simulink model "Simulink_Model"  (R2021a)
settings: Solver=VariableStepAuto  StartTime=0.0  StopTime=inf  FixedStep=1  RelTol=1e-3
model workspace (MAT data in the model file):
  M = 1200
  R = 1
libraries: pid_lib x1
settings Model: EnablePacing=on  Creator=matteopenlington  LastModifiedBy=matteopenlington
settings DebuggingCC: UnderSpecifiedDimensionMsg=warning

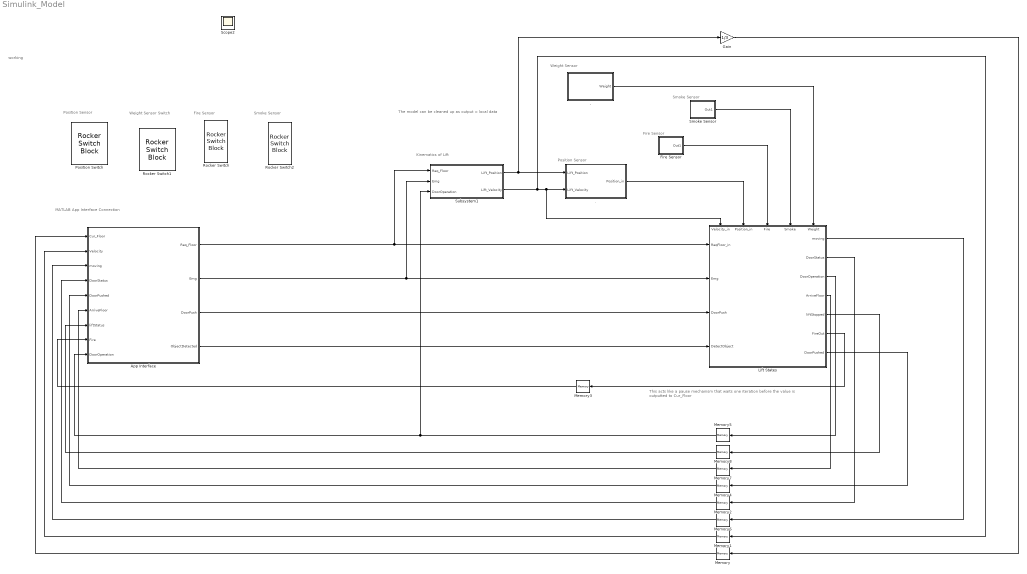
== system Simulink_Model ==
  note: working
  note: MATLAB App Interface Connection
  note: Fire Sensor
  note: Smoke Sensor
  note: Kinematics of Lift
  note: The model can be cleaned up as output = local data
  note: This acts like a pause mechanism that
      | waits one iteration before the value is
      | outputted to Cur_Floor
  note: Weight Sensor Switch
  note: Weight Sensor
  note: Position Sensor
  note: Position Sensor
  note: Fire Sensor
  note: Smoke Sensor
  , : Subsystem
  . : Subsystem
  App Interface : Stateflow chart  TreatAsAtomicUnit=on
      settings: PortSchema="{\"entries\":[{\"content\":{\"sides\":[{\"content\":{\"connectorIds\":[\"In1\",\"In2\",\"In6\",\"In3\",\"In4\",\"In7\",\"In9\",\"In8\",\"In5\"]},\"type\":\"ConnectorPlacement.EquallySpacedRectSide\",\"uuid\":\"ef86dee1-50cd-47ea-bc75-e3c16101b464\"},{\"content\":{\"connectorIds\":[\"Out1\",\"Out2\",\"Out3\",\"Out4\"],\"side\":\"RIGHT\"},\"type\":\"ConnectorPlacement.EquallySpacedRectSide\",\"uuid\":\"2ba459ed-9838-4da4-8149-392158b3da7c\"},{\"content\":{\"connectorIds\":[],\"side\":\"TOP\"},\"type\":\"ConnectorPlacement.EquallySpacedRectSide\",\"uuid\":\"d04a1450-e40a-42c5-8ca5-ab8bc8570c42\"}]},\"type\":\"ConnectorPlacement.EquallySpacedConnector\",\"uuid\":\"548c1efd-1acc-447b-a5db-88314a01fdab\"}],\"packageUris\":[\"http://schema.mathworks.com/mf0/Connector/R2020b\"],\"version\":\"1.0\"}"
  Fire Sensor : Subsystem
  Gain : Gain  Gain=1/3
  Lift States : Stateflow chart  TreatAsAtomicUnit=on
      settings: PortSchema="{\"entries\":[{\"content\":{\"sides\":[{\"content\":{\"connectorIds\":[\"In1\",\"In5\",\"In6\",\"In7\"]},\"type\":\"ConnectorPlacement.EquallySpacedRectSide\",\"uuid\":\"bd67e075-ced7-4894-beb9-3d24b34d513a\"},{\"content\":{\"connectorIds\":[\"Out1\",\"Out2\",\"Out4\",\"Out5\",\"Out6\",\"Out7\",\"Out3\"],\"side\":\"RIGHT\"},\"type\":\"ConnectorPlacement.EquallySpacedRectSide\",\"uuid\":\"62974800-2f1d-440c-84a5-b13d0b321f49\"},{\"content\":{\"connectorIds\":[\"In9\",\"In8\",\"In3\",\"In4\",\"In2\"],\"side\":\"TOP\"},\"type\":\"ConnectorPlacement.EquallySpacedRectSide\",\"uuid\":\"b0ebe389-7aaa-432d-aca6-247e3589a149\"}]},\"type\":\"ConnectorPlacement.EquallySpacedConnector\",\"uuid\":\"bed4184c-0ba6-4939-b370-ce80092994a7\"}],\"packageUris\":[\"http://schema.mathworks.com/mf0/Connector/R2020b\"],\"version\":\"1.0\"}"
  Memory{,1..8} (9 alike) : Memory
  Position Switch : RockerSwitchBlock
      settings: Values={{'Off', 'On'}, [0 1]}
  Rocker Switch : RockerSwitchBlock
      settings: Values={{'Off', 'On'}, [0 1]}
  Rocker Switch1 : RockerSwitchBlock
      settings: Values={{'Off', 'On'}, [0 1]}
  Rocker Switch2 : RockerSwitchBlock
      settings: Values={{'Off', 'On'}, [0 1]}
  Smoke Sensor : Subsystem
  Subsystem1 : Subsystem
  Scope2 : Scope
  wires:
  ./1(Position_in) -> Lift States/8(Position_in)
  Memory2/1 -> App Interface/3(DoorStatus)
  App Interface/4(ObjectDetected) -> Lift States/7(DetectObject)
  Memory4/1 -> App Interface/4(DoorPushed)
  Lift States/4(DoorOperation) -> Memory5/1
  Lift States/3(DoorPushed) -> Memory4/1
  Memory/1 -> App Interface/1(Cur_Floor)
  Memory6/1 -> App Interface/6(moving)
  Lift States/5(ArriveFloor) -> Memory7/1
  Subsystem1/1(Lift_Position) -> ./1(Lift_Position), Gain/1
  Subsystem1/2(Lift_Velocity) -> ./2(Lift_Velocity), Lift States/9(Velocity_in), Memory1/1
  Lift States/2(DoorStatus) -> Memory2/1
  Memory5/1 -> Subsystem1/3(DoorOperation), App Interface/5(DoorOperation)
  Lift States/1(moving) -> Memory6/1
  App Interface/3(DoorPush) -> Lift States/6(DoorPush)
  ,/1(Weight) -> Lift States/2(Weight)
  Memory1/1 -> App Interface/2(Velocity)
  Gain/1 -> Memory/1
  App Interface/2(Emg) -> Subsystem1/2(Emg), Lift States/5(Emg)
  App Interface/1(Req_Floor) -> Subsystem1/1(Req_Floor), Lift States/1(ReqFloor_in)
  Memory7/1 -> App Interface/7(ArriveFloor)
  Fire Sensor/1(Out1) -> Lift States/3(Fire)
  Smoke Sensor/1(Out1) -> Lift States/4(Smoke)
  Lift States/6(liftStopped) -> Memory8/1
  Memory8/1 -> App Interface/9(liftStatus)
  Lift States/7(FireOut) -> Memory3/1
  Memory3/1 -> App Interface/8(Fire)

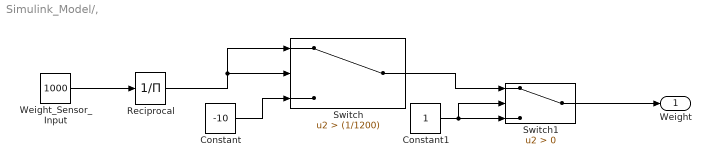
== system Simulink_Model/, ==
  Constant : Constant  Value=-10
  Constant1 : Constant
  Reciprocal : Product  Inputs=/
  Switch : Switch  Criteria=u2 > Threshold  Threshold=(1/1200)
  Switch1 : Switch  Criteria=u2 > Threshold
  Weight_Sensor_Input : Constant  Value=1000
  Weight : Outport
  wires:
  Weight_Sensor_Input/1 -> Reciprocal/1
  Switch/1 -> Switch1/1
  Constant/1 -> Switch/3
  Constant1/1 -> Switch1/3, Switch1/2
  Switch1/1 -> Weight/1
  Reciprocal/1 -> Switch/1, Switch/2

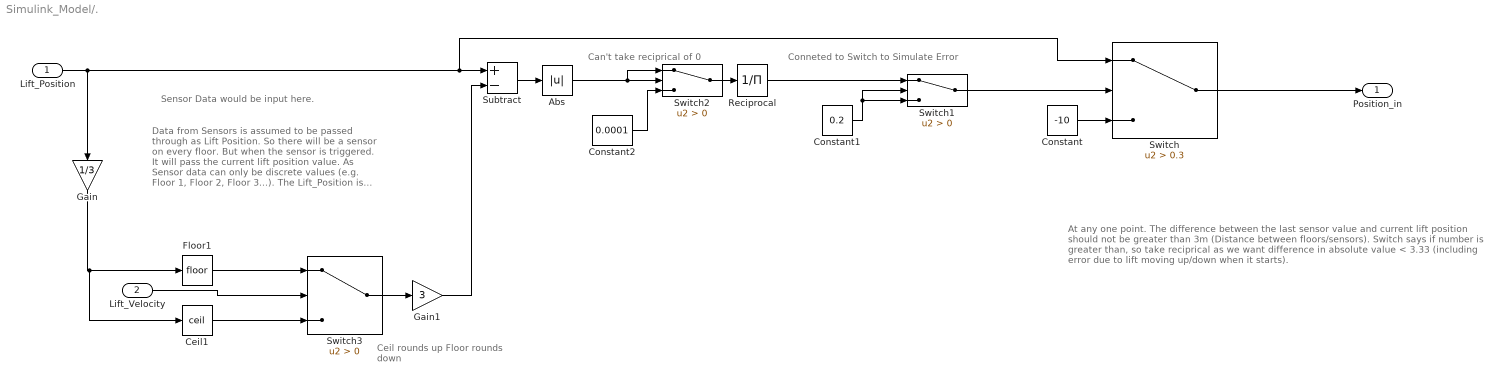
== system Simulink_Model/. ==
  note: Can't take reciprical of 0
  note: At any one point. The difference between the last sensor value and current lift position should not be greater than 3m (Distance between floors/sensors).
      |
      | Switch says if number is greater than, so take reciprical as we want difference in absolute value < 3.33 (including error due to lift moving up/down when it starts).
  note: Ceil rounds up
      | Floor rounds down
  note: Data from Sensors is assumed to be passed through as Lift Position. So there will be a sensor on every floor. But when the sensor is triggered. It will pass the current lift position value.
      |
      | As Sensor data can only be discrete values (e.g. Floor 1, Floor 2, Floor 3...). The Lift_Position is rounded to the integer according to whether velocity is up or down, as the opposite will be where the last stop was.
  note: Sensor Data would be input here.
  note: Conneted to Switch to Simulate Error
  Lift_Position : Inport
  Lift_Velocity : Inport  Port=2
  Abs : Abs
  Ceil1 : Rounding  Operator=ceil
  Constant : Constant  Value=-10
  Constant1 : Constant  Value=0.2
  Constant2 : Constant  Value=0.0001
  Floor1 : Rounding
  Gain : Gain  Gain=1/3
  Gain1 : Gain  Gain=3
  Reciprocal : Product  Inputs=/
  Subtract : Sum  Inputs=+-
  Switch : Switch  Criteria=u2 > Threshold  Threshold=0.3
  Switch1 : Switch  Criteria=u2 > Threshold
  Switch2 : Switch  Criteria=u2 > Threshold
  Switch3 : Switch  Criteria=u2 > Threshold
  Position_in : Outport
  wires:
  Lift_Position/1 -> Subtract/1, Switch/1, Gain/1
  Subtract/1 -> Abs/1
  Constant/1 -> Switch/3
  Switch/1 -> Position_in/1
  Switch1/1 -> Switch/2
  Abs/1 -> Switch2/1, Switch2/2
  Constant1/1 -> Switch1/3, Switch1/2
  Lift_Velocity/1 -> Switch3/2
  Switch3/1 -> Gain1/1
  Floor1/1 -> Switch3/1
  Ceil1/1 -> Switch3/3
  Gain/1 -> Floor1/1, Ceil1/1
  Gain1/1 -> Subtract/2
  Constant2/1 -> Switch2/3
  Switch2/1 -> Reciprocal/1
  Reciprocal/1 -> Switch1/1

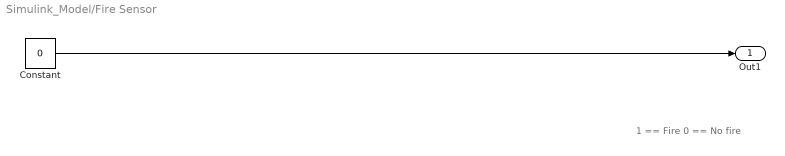
== system Simulink_Model/Fire Sensor ==
  note: 1 == Fire
      | 0 == No fire
  Constant : Constant  Value=0
  Out1 : Outport
  wires:
  Constant/1 -> Out1/1

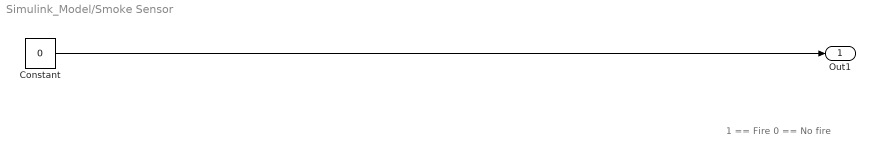
== system Simulink_Model/Smoke Sensor ==
  note: 1 == Fire
      | 0 == No fire
  Constant : Constant  Value=0
  Out1 : Outport
  wires:
  Constant/1 -> Out1/1

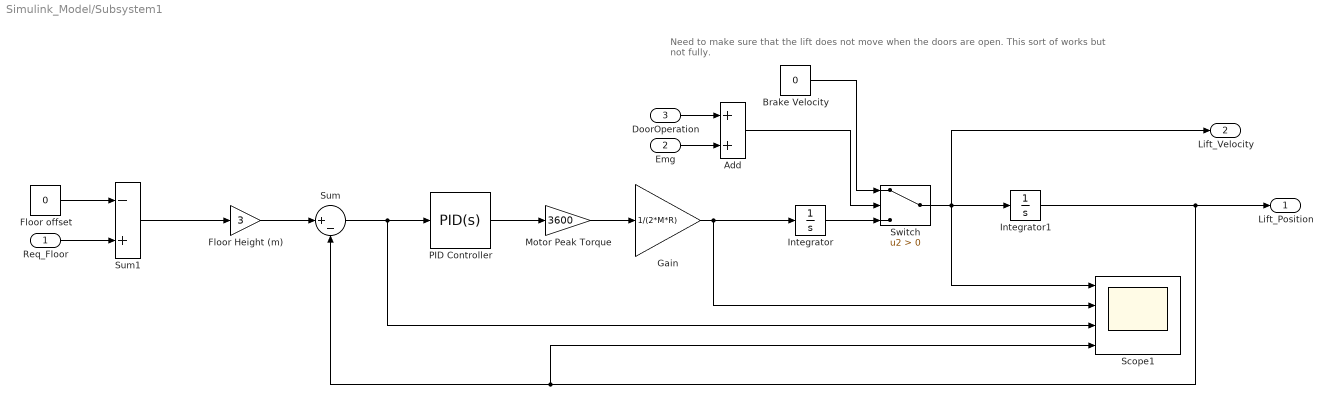
== system Simulink_Model/Subsystem1 ==
  note: Need to make sure that the lift does not move when the doors are open. This sort of works but not fully.
  Req_Floor : Inport
  Emg : Inport  Port=2
  DoorOperation : Inport  Port=3
  Add : Sum
  Brake Velocity : Constant  Value=0
  Floor Height (m) : Gain  Gain=3
  Floor offset : Constant  Value=0
  Gain : Gain  Gain=1/(2*M*R)
  Integrator : Integrator
  Integrator1 : Integrator
  Motor Peak Torque : Gain  Gain=3600
  PID Controller : pid_lib/PID Controller  Controller=PID  Form=Parallel  TimeDomain=Continuous-time  UseExternalTs=off  SampleTime=-1  IntegratorMethod=Forward Euler  FilterMethod=Forward Euler  ControllerParametersSource=internal  P=1  I=0  D=2  UseFilter=on  N=5.45  TunerSelectOption=Transfer Function Based (PID Tuner App)  InitialConditionSource=internal  InitialConditionForIntegrator=0  InitialConditionForFilter=0  DifferentiatorICPrevScaledInput=0  ExternalReset=none  TrackingMode=off  Kt=1  LimitOutput=on  SatLimitsSource=internal  UpperSaturationLimit=1  LowerSaturationLimit=-1  LinearizeAsGain=on  AntiWindupMode=none  Kb=1  POutMin=[]  POutMax=[]  IOutMin=[]  IOutMax=[]  DOutMin=[]  DOutMax=[]  NOutMin=[]  NOutMax=[]  SumOutMin=[]  SumOutMax=[]  SaturationOutMin=[]  SaturationOutMax=[]  PParamMin=[]  PParamMax=[]  IParamMin=[]  IParamMax=[]  DParamMin=[]  DParamMax=[]  NParamMin=[]  NParamMax=[]  KbParamMin=[]  KbParamMax=[]  KtParamMin=[]  KtParamMax=[]  KbOutMin=[]  KbOutMax=[]  KtOutMin=[]  KtOutMax=[]  IntegratorOutMin=[]  IntegratorOutMax=[]  FilterOutMin=[]  FilterOutMax=[]  SumI1OutMin=[]  SumI1OutMax=[]  SumI2OutMin=[]  SumI2OutMax=[]  SumI3OutMin=[]  SumI3OutMax=[]  SumI4OutMin=[]  SumI4OutMax=[]  SumDOutMin=[]  SumDOutMax=[]  DifferentiatorOutMin=[]  DifferentiatorOutMax=[]  FilterDiffOutCoefMin=[]  FilterDiffOutCoefMax=[]  ReciprocalOutMin=[]  ReciprocalOutMax=[]  SumDenOutMin=[]  SumDenOutMax=[]  SumNumOutMin=[]  SumNumOutMax=[]  DivideOutMin=[]  DivideOutMax=[]  UdiffTsProdOutMin=[]  UdiffTsProdOutMax=[]  NTsProdOutMin=[]  NTsProdOutMax=[]  UintegralTsProdOutMin=[]  UintegralTsProdOutMax=[]  UngainTsProdOutMin=[]  UngainTsProdOutMax=[]  IntegratorContinuousStateAttributes=''  IntegratorStateMustResolveToSignalObject=off  IntegratorRTWStateStorageClass=Auto  FilterContinuousStateAttributes=''  FilterStateMustResolveToSignalObject=off  FilterRTWStateStorageClass=Auto  ParallelPVariant=InternalParameters  IdealPVariant=Disabled  IVariant=InternalParameters  DVariant=InternalParameters  IntegratorVariant=Continuous  SatVariant=Enabled  AWVariant=Passthrough  PCopyVariant=Disabled  TRVariant=Disabled  FdbkBlocksVariant=Forward  IdealPFdbkVariant=Disabled  SatFdbkVariant=Disabled  DerivativeFilterVariant=ContFilter  NVariant=InternalParameters  NCopyVariant=Disabled  FilterICVariant=InternalICsFilter  IntegratorICVariant=InternalICs  ExternalResetVariant=Disabled  TRSumVariant=Passthrough  SumFdbkVariant=Disabled  SumVariant=Sum_PID  TsampFilterVariant=InternalTs  TsampNgainVariant=Passthrough  TsampIntegralVariant=Passthrough  ExternalSaturationOutDataTypeStr=Inherit: Same as second input
  Scope1 : Scope  NumInputPorts=4
  Sum : Sum  Inputs=|+-
  Sum1 : Sum  Inputs=-+
  Switch : Switch  Criteria=u2 > Threshold
  Lift_Position : Outport
  Lift_Velocity : Outport  Port=2
  wires:
  Req_Floor/1 -> Sum1/2
  Gain/1 -> Scope1/2, Integrator/1
  Sum/1 -> Scope1/3, PID Controller/1
  PID Controller/1 -> Motor Peak Torque/1
  Floor Height (m)/1 -> Sum/1
  Sum1/1 -> Floor Height (m)/1
  Integrator/1 -> Switch/3
  Integrator1/1 -> Lift_Position/1, Scope1/4, Sum/2
  Motor Peak Torque/1 -> Gain/1
  Floor offset/1 -> Sum1/1
  Switch/1 -> Scope1/1, Lift_Velocity/1, Integrator1/1
  Brake Velocity/1 -> Switch/1
  Emg/1 -> Add/2
  DoorOperation/1 -> Add/1
  Add/1 -> Switch/2

== stateflow chart Simulink_Model/App Interface ==
  state InterfaceFromApp
    en:
    coder.extrinsic('AppWSimulink', 'updateCounter', 'Emergency', 'DoorOperationReq', 'updateDoorStatus', 'CallDirection', 'liftCall', 'DetectObject', 'liftStopped', 'FireFnc', 'checkPassengerMatrix');
    app = AppWSimulink(this);
    initialiseData();
    Emergency(app,Emg);
    DoorOperationReq(app, DoorPush);
    %liftCall(app, Velocity, Cur_Floor);
    du:
    if hasChanged(Cur_Floor)
    updateCounter(app, Cur_Floor, moving, DoorOperation);
    end
    if abs(Req_Floor - Cur_Floor) < 0.1
    updateDoorStatus(app,DoorStatus, Cur_Floor, ArriveFloor);
    end
    if (Emg == 1)
    Reset;
    end
    if DoorPushed == 1
    DoorPush = -2;
    end
    if DoorOperation == 0
    end
    DetectObject(app);
    if DoorOperation == 1
    Req_Floor = Cur_Floor;
    end
    if liftStatus == 1 && ifRequested == 1
    liftStopped(app);
    end
    if Fire == 1
    %FireFnc(app)
    end
    if moving == 1
    ifRequested = 0;
    end
    % checkPassengerMatrix(app)
    liftDesination = Req_Floor;
    state initialiseData [function]
      (default) -> (junction 12) : {
          | %CurFloor = 0;
          | Req_Floor = 1;
          | Emg = 0;
          | DoorPush =-2;
          | ObjectDetected =0;
          | ifRequested = 0;
          | }
    state Reset [function]
      (default) -> (junction 119) : {
          | Req_Floor = Cur_Floor;
          | DoorPush =3;
          | }
  (default) -> InterfaceFromApp
  data: app local; Cur_Floor input; Req_Floor output; Emg output; Velocity input; DoorPush output; DoorStatus input; ObjectDetected output; DoorPushed input; DoorOperation input; moving input; ArriveFloor input; Fire input; liftStatus input; liftDesination local; ifRequested local

== stateflow chart Simulink_Model/Lift States ==
  state No_Error2
    en:
    initialiseData;
    state initialiseData [function]
      (default) -> (junction 330) : {door = 0;
          | doorClose = 0;
          | hasOpened = 1;
          | ArriveFloor = 0;
          | DoorStatus = 3;
          | DoorOperation = 0;
          | DoorPushed = 0;
          | }
    state Motion [group]
      state MovingUp
        entry:
        moving = 1;
        liftStopped = 0;
        hasOpened =0;
        exit:
        moving = 0;
      state MovingDown
        entry:
        moving = 2;
        liftStopped = 0;
        hasOpened = 0;
        exit:
        moving =0;
    state Not_Moving
      entry:
      Cur_Floor;
      NxtFloor;
      liftStopped = 1;
      state NxtFloor [function]
        (default) -> (junction 212)
        (junction 212) -> (junction 213) [order 1] : [isempty(ReqFloor_in)]{ReqFloor = -10}
        (junction 212) -> (junction 214) [order 2] : {ReqFloor = ReqFloor_in;}
        (junction 213) -> (junction 215)
        (junction 214) -> (junction 215)
      state Idle
        en:
      state Doors
        note: Value of door isn't always 0 or 1
            |
            | Object Detection is always running whilst open. Value is simulated through app interface button.
        state OpOpening [function]
          note: If the door movement was simulated that value would end up being exactly 0 or 1. Because of step iterations you end up with 1.1 and -0.1. But the transitions account for this.
          (default) -> (junction 231) : [door <= 1]{door = door + 0.1;}
        state DoorOpening
          en:
          door = 0;
          doorClose = 0;
          DoorStatus = 0;
          du:
          OpOpening;
        state OpClosing [function]
          (default) -> (junction 244) : {door = door - 0.1;}
        state DoorClosing
          en:
          DoorStatus = 2;
          DoorPushed = 0;
          du:
          OpClosing;
        state DoorOpen
          entry:
          DoorStatus = 1;
          hasOpened = 1;
        state DoorClosed
          entry:
          DoorStatus =3;
          pause(2);
          doorClose = 1;
        (junction 318) -> DoorOpening
        DoorClosing -> (junction 318) [order 1] : [DetectObject == 1]
        (junction 321) -> DoorOpening
        DoorClosing -> (junction 321) [order 2] : [DoorPush == 0]{DoorPushed = 1;}
        DoorOpening -> DoorOpen : [door >= 1]{DoorPushed = 0;}
        DoorOpen -> DoorClosing [order 2] : [DoorPush == 1 && DetectObject == 0]{DoorPushed = 1;}
        DoorClosing -> DoorClosed [order 3] : [door <= 0]
        DoorOpen -> DoorClosing [order 1] : after(2,sec)[DetectObject == 0]
      (default) -> Idle
      Idle -> DoorOpening [order 1] : [ (ReqFloor - CurFloor)<0.01 && hasOpened == 0]{DoorOperation =1;, ArriveFloor=1;}
    state Cur_Floor [function]
      (default) -> (junction 279) : {CurFloor = (Position_in/3);}
    note: Set DoorPush == -2 because it has been completed. But don't want to set ObjectDetected == 0 because we need to run again and make sure there are no objects in the way.
    (default) -> Not_Moving
    Not_Moving -> MovingUp [order 1] : [Velocity_in > 0.2 && DoorOperation == 0]
    MovingUp -> Not_Moving : [abs(Velocity_in) < 0.01]
    Idle -> (junction 192) [order 2]
    (junction 192) -> (junction 193)
    Not_Moving -> MovingDown [order 2] : [Velocity_in < -0.2 && DoorOperation == 0]
    (junction 193) -> Not_Moving : after(1,sec)
    (junction 194) -> (junction 193)
    MovingDown -> Not_Moving : [abs(Velocity_in) < 0.01]
    Doors -> (junction 194) : [doorClose == 1]{DoorOperation = 0;, ArriveFloor = 0;}
  state Error_States
    en:
    state Emergency
      en:
      DoorStatus = 3;
      hasOpened = 0;
      moving = 0;
    state Position_Sensor
      en:
      DoorStatus = 0;
      hasOpened = 0;
      moving = 0;
    state Weight_Limit
      % call to intercom to say passengers need to get off.
      en:
      DoorStatus = 0;
      hasOpened = 0;
      moving = 0;
    state Fire
      en:
      DoorStatus = 3;
      hasOpened = 0;
      moving = 0;
      FireOut == 1;
    state Smoke
      en:
      DoorStatus = 3;
      hasOpened = 0;
      moving = 0;
  (default) -> No_Error2
  No_Error2 -> Emergency [order 1] : [Emg == 1]
  Emergency -> No_Error2 : [Emg  == 0]
  No_Error2 -> Position_Sensor [order 2] : [Position_in == -10]
  Position_Sensor -> No_Error2 : [Position_in~= -10]
  No_Error2 -> Weight_Limit [order 3] : [Weight == -10]
  Weight_Limit -> No_Error2 : [Weight ~= -10]
  No_Error2 -> Fire [order 4] : [Fire == 1]
  Fire -> No_Error2 : [Fire == 0]
  No_Error2 -> Smoke [order 5] : [Smoke == 1]
  Smoke -> No_Error2 : [Smoke == 0]
  data: CurFloor local; ReqFloor_in input; Weight input; Fire input; Smoke input; ReqFloor local; Emg input; moving output =0; DoorPush input; DetectObject input; door local; DoorStatus output =0; DoorPushed output =0; hasOpened local; doorClose local; Position_in input; Velocity_in input; Passengers local; DoorOperation output =0; ArriveFloor output =0; liftStopped output =0; FireOut output =0
